simulink library "PDECharactLib"  (R2019a)
settings: Solver=VariableStepAuto  StartTime=0.0  StopTime=10.0  RelTol=1e-3
settings Model: Creator=User  LastModifiedBy=kc5492

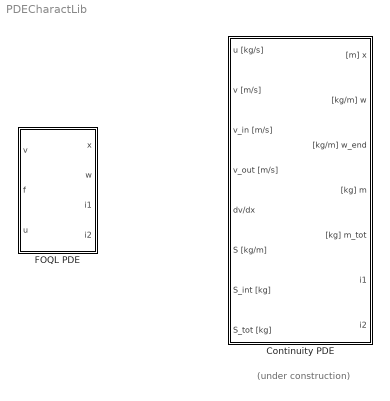
== system PDECharactLib ==
  note: (under construction)
  Continuity PDE : Subsystem  mask(First-order quasilinear PDE solver){ell=1, Nmax=100, x0=0:0.1:1, w0=1:-0.1:0, m0=0.095:-0.01:0.005, initM_tot=0, initX=0, initW=0, initM=0, dx=0.1, dw=0.1, dt=0.1, crossing_tol=1e-11, overflow_err=off}
      mask prompts: ell "Domain length (L)"; Nmax "Maximum number of characteristics (Nmax)"; x0 "x-values"; w0 "w-values"; m0 "m-values"; initM_tot "total mass"; initX "(hidden) Full initial x"; initW "(hidden) Full initial w"; initM "(hidden) Full initial m"; dx "∆x"; dw "∆w"; dt "∆t"; crossing_tol "Tolerance for crossing characteristics"; overflow_err "Terminate on overflow"
      mask help:
      | Implementation of the method of characteristics for the first-order quasilinear PDE
      |
      | 	∂w(t, x)/∂t + v(t, x) ∂w(t, x)/∂x = f(t, x),    t ≥ 0,    x ∈ [0, L],
      | 	w(0, x) = w0(x),
      | 	w(t, 0) = u(t).
      |
      | The functions v, f, and u are provided through the inputs and can also depend on variables other than time.
      |
      | The number of characteristics to be integrated simultaneously is limited by Nmax. The current number of characteristics is output through the port N.
      |
      | Initial state function w0(x) is defined by its grid values (x, w) which also define the initial set of characteristics. The vector of x-values should be non-decreasing and span from 0 to L. The vector of w-values should be the same length as x-values.
      |
      | If the latest characteristic was created at time t0 and currently passes through the point (x, w) then new characteristic is created at the boundary x = 0 if at least one of the conditions is satisfied:
      |     • x > ∆x,
      |     • |w - u(t)| > ∆w,
      |     • t - t0 > ∆t.
      |
      | Error is thrown when two characteristics intersect with overlap more than that defined as "Tolerance for crossing characteristics" or when the flag "Terminate on overflow" is set and the number of characteristics exceeds Nmax.
      mask init:
      | initX = [x0, zeros(1, Nmax-length(x0))];
      | initW = [w0, zeros(1, Nmax-length(w0))];
      | initM = [0, m0, zeros(1, Nmax-length(m0)-1)];
      mask DialogControl Container4 Prompt: Initial state
      mask DialogControl Container3 Prompt: Conditions for creating a new characteristic
  FOQL PDE : Subsystem  mask(First-order quasilinear PDE solver){ell=1, Nmax=100, x0=0:0.1:1, w0=(0:0.1:1).^2, initX=0, initW=0, dx=0.1, dw=0.1, dt=0.1, crossing_tol=1e-11, overflow_err=off}
      mask prompts: ell "Domain length (L)"; Nmax "Maximum number of characteristics (Nmax)"; x0 "x-values"; w0 "w-values"; initX "(hidden) Full initial x"; initW "(hidden) Full initial w"; dx "∆x"; dw "∆w"; dt "∆t"; crossing_tol "Tolerance for crossing characteristics"; overflow_err "Terminate on overflow"
      mask help:
      | Implementation of the method of characteristics for the first-order quasilinear PDE
      |
      | 	∂w(t, x)/∂t + v(t, x) ∂w(t, x)/∂x = f(t, x),    t ≥ 0,    x ∈ [0, L],
      | 	w(0, x) = w0(x),
      | 	w(t, 0) = u(t).
      |
      | The functions v, f, and u are provided through the inputs and can also depend on variables other than time.
      |
      | The number of characteristics to be integrated simultaneously is limited by Nmax. The current number of characteristics is output through the port N.
      |
      | Initial state function w0(x) is defined by its grid values (x, w) which also define the initial set of characteristics. The vector of x-values should be non-decreasing and span from 0 to L. The vector of w-values should be the same length as x-values.
      |
      | If the latest characteristic was created at time t0 and currently passes through the point (x, w) then new characteristic is created at the boundary x = 0 if at least one of the conditions is satisfied:
      |     • x > ∆x,
      |     • |w - u(t)| > ∆w,
      |     • t - t0 > ∆t.
      |
      | Error is thrown when two characteristics intersect with overlap more than that defined as "Tolerance for crossing characteristics" or when the flag "Terminate on overflow" is set and the number of characteristics exceeds Nmax.
      mask init:
      | initX = [x0, zeros(1, Nmax-length(x0))];
      | initW = [w0, zeros(1, Nmax-length(w0))];
      mask DialogControl Container4 Prompt: Initial state
      mask DialogControl Container3 Prompt: Conditions for creating a new characteristic

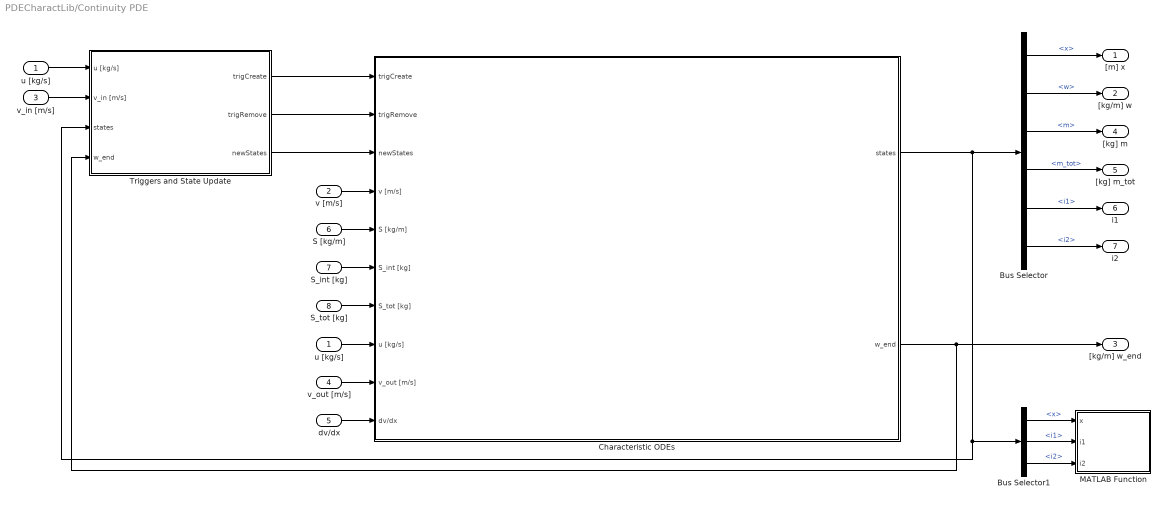
== system PDECharactLib/Continuity PDE ==
  u [kg/s] : Inport
  v [m/s] : Inport  Port=2
  v_in [m/s] : Inport  Port=3
  v_out [m/s] : Inport  Port=4
  dv/dx : Inport  Port=5
  S [kg/m] : Inport  Port=6
  S_int [kg] : Inport  Port=7
  S_tot [kg] : Inport  Port=8
  " u [kg/s] " : InportShadow
  Bus Selector : BusSelector  OutputSignals=x,w,m,m_tot,i1,i2
  Bus Selector1 : BusSelector  OutputSignals=x,i1,i2
  Characteristic ODEs : Subsystem
  MATLAB Function : MATLAB Function  TreatAsAtomicUnit=on
  Triggers and State Update : Subsystem
  "[m] x" : Outport
  "[kg/m] w" : Outport  Port=2
  "[kg/m] w_end" : Outport  Port=3
  "[kg] m" : Outport  Port=4
  "[kg] m_tot" : Outport  Port=5
  i1 : Outport  Port=6
  i2 : Outport  Port=7
  wires:
  u [kg/s]/1 -> Triggers and State Update/1(u [kg/s])
  v [m/s]/1 -> Characteristic ODEs/4(v [m/s])
  Triggers and State Update/1(trigCreate) -> Characteristic ODEs/1(trigCreate)
  Triggers and State Update/2(trigRemove) -> Characteristic ODEs/2(trigRemove)
  S [kg/m]/1 -> Characteristic ODEs/5(S [kg/m])
  S_int [kg]/1 -> Characteristic ODEs/6(S_int [kg])
  S_tot [kg]/1 -> Characteristic ODEs/7(S_tot [kg])
  " u [kg/s] "/1 -> Characteristic ODEs/8(u [kg/s])
  v_out [m/s]/1 -> Characteristic ODEs/9(v_out [m/s])
  dv/dx/1 -> Characteristic ODEs/10(dv/dx)
  Triggers and State Update/3(newStates) -> Characteristic ODEs/3(newStates)
  Characteristic ODEs/1(states) -> Triggers and State Update/3(states), Bus Selector1/1, Bus Selector/1
  Characteristic ODEs/2(w_end) -> Triggers and State Update/4(w_end), "[kg/m] w_end"/1
  Bus Selector/1 -> "[m] x"/1  "<x>"
  Bus Selector/2 -> "[kg/m] w"/1  "<w>"
  Bus Selector/3 -> "[kg] m"/1  "<m>"
  Bus Selector/4 -> "[kg] m_tot"/1  "<m_tot>"
  Bus Selector/5 -> i1/1  "<i1>"
  Bus Selector/6 -> i2/1  "<i2>"
  Bus Selector1/1 -> MATLAB Function/1(x)  "<x>"
  Bus Selector1/2 -> MATLAB Function/2(i1)  "<i1>"
  Bus Selector1/3 -> MATLAB Function/3(i2)  "<i2>"
  v_in [m/s]/1 -> Triggers and State Update/2(v_in [m/s])

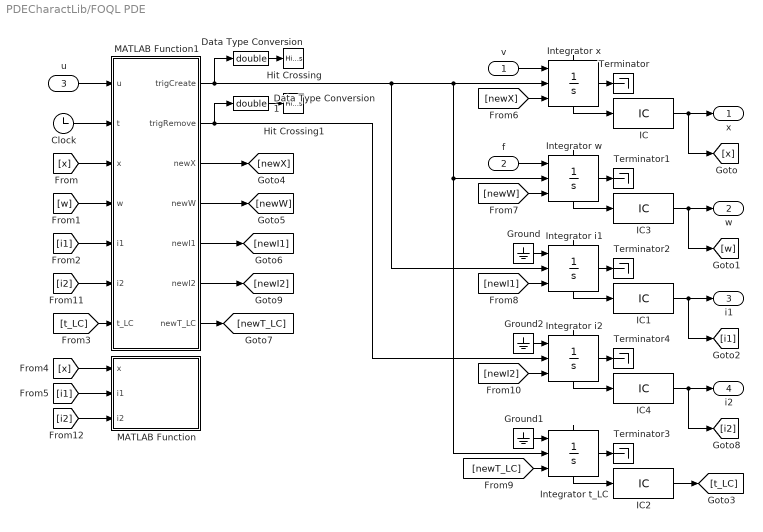
== system PDECharactLib/FOQL PDE ==
  v : Inport
  f : Inport  Port=2
  u : Inport  Port=3
  Clock : Clock
  Data Type Conversion : DataTypeConversion  OutDataTypeStr=double
  Data Type Conversion1 : DataTypeConversion  OutDataTypeStr=double
  Ground : Ground
  Ground1 : Ground
  Ground2 : Ground
  Hit Crossing : HitCross  ShowOutputPort=off
  Hit Crossing1 : HitCross  ShowOutputPort=off
  IC : InitialCondition  Value=initX
  IC1 : InitialCondition
  IC2 : InitialCondition  Value=0
  IC3 : InitialCondition  Value=initW
  IC4 : InitialCondition  Value=length(x0)
  Integrator i1 : Integrator  ExternalReset=level hold  InitialConditionSource=external  InitialCondition=[length(x0); 0]  ShowStatePort=on
  Integrator i2 : Integrator  ExternalReset=level hold  InitialConditionSource=external  InitialCondition=[length(x0); 0]  ShowStatePort=on
  Integrator t_LC : Integrator  ExternalReset=level hold  InitialConditionSource=external  InitialCondition=[length(x0); 0]  ShowStatePort=on
  Integrator w : Integrator  ExternalReset=level hold  InitialConditionSource=external  ShowStatePort=on
  Integrator x : Integrator  ExternalReset=level hold  InitialConditionSource=external  ShowStatePort=on
  MATLAB Function : MATLAB Function  TreatAsAtomicUnit=on
  MATLAB Function1 : MATLAB Function  TreatAsAtomicUnit=on
  Terminator{,1..4} (5 alike) : Terminator
  x : Outport
  w : Outport  Port=2
  i1 : Outport  Port=3
  i2 : Outport  Port=4
  wires:
  Integrator x/State -> IC/1
  u/1 -> MATLAB Function1/1(u)
  Clock/1 -> MATLAB Function1/2(t)
  Integrator i1/State -> IC1/1
  Integrator t_LC/State -> IC2/1
  MATLAB Function1/1(trigCreate) -> Integrator w/2, Integrator t_LC/2, Integrator x/2, Integrator i1/2, Data Type Conversion/1
  Data Type Conversion/1 -> Hit Crossing/1
  Data Type Conversion1/1 -> Hit Crossing1/1
  IC/1 -> x/1, [x]
  IC3/1 -> w/1, [w]
  Integrator w/State -> IC3/1
  v/1 -> Integrator x/1
  f/1 -> Integrator w/1
  IC1/1 -> i1/1, [i1]
  Ground/1 -> Integrator i1/1
  Ground1/1 -> Integrator t_LC/1
  Integrator x/1 -> Terminator/1
  Integrator w/1 -> Terminator1/1
  Integrator i1/1 -> Terminator2/1
  Integrator t_LC/1 -> Terminator3/1
  IC2/1 -> [t_LC]
  MATLAB Function1/3(newX) -> [newX]
  MATLAB Function1/4(newW) -> [newW]
  MATLAB Function1/5(newI1) -> [newI1]
  MATLAB Function1/7(newT_LC) -> [newT_LC]
  MATLAB Function1/2(trigRemove) -> Integrator i2/2, Data Type Conversion1/1
  [newT_LC] -> Integrator t_LC/3
  [newX] -> Integrator x/3
  [newW] -> Integrator w/3
  [newI1] -> Integrator i1/3
  [x] -> MATLAB Function/1(x)
  [i1] -> MATLAB Function/2(i1)
  [t_LC] -> MATLAB Function1/7(t_LC)
  [i1] -> MATLAB Function1/5(i1)
  [w] -> MATLAB Function1/4(w)
  [x] -> MATLAB Function1/3(x)
  [newI2] -> Integrator i2/3
  Integrator i2/1 -> Terminator4/1
  IC4/1 -> [i2], i2/1
  Integrator i2/State -> IC4/1
  Ground2/1 -> Integrator i2/1
  [i2] -> MATLAB Function1/6(i2)
  [i2] -> MATLAB Function/3(i2)
  MATLAB Function1/6(newI2) -> [newI2]

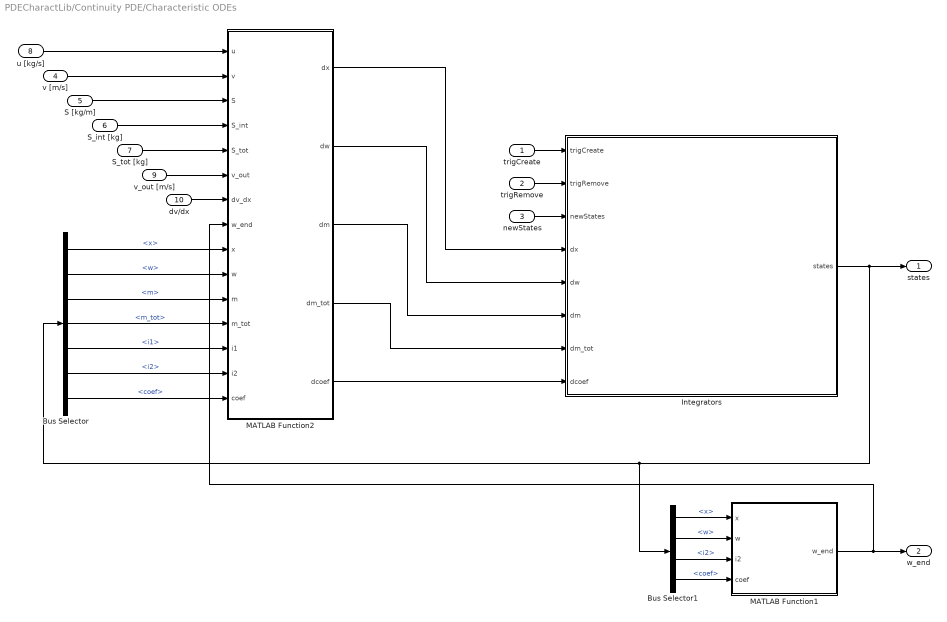
== system PDECharactLib/Continuity PDE/Characteristic ODEs ==
  trigCreate : Inport
  trigRemove : Inport  Port=2
  newStates : Inport  Port=3
  v [m/s] : Inport  Port=4
  S [kg/m] : Inport  Port=5
  S_int [kg] : Inport  Port=6
  S_tot [kg] : Inport  Port=7
  u [kg/s] : Inport  Port=8
  v_out [m/s] : Inport  Port=9
  dv/dx : Inport  Port=10
  Bus Selector : BusSelector  OutputSignals=x,w,m,m_tot,i1,i2,coef
  Bus Selector1 : BusSelector  OutputSignals=x,w,i2,coef
  Integrators : Subsystem
  MATLAB Function1 : MATLAB Function  TreatAsAtomicUnit=on
  MATLAB Function2 : MATLAB Function  TreatAsAtomicUnit=on
  states : Outport
  w_end : Outport  Port=2
  wires:
  S [kg/m]/1 -> MATLAB Function2/3(S)
  v_out [m/s]/1 -> MATLAB Function2/6(v_out)
  u [kg/s]/1 -> MATLAB Function2/1(u)
  S_tot [kg]/1 -> MATLAB Function2/5(S_tot)
  trigRemove/1 -> Integrators/2(trigRemove)
  dv/dx/1 -> MATLAB Function2/7(dv_dx)
  S_int [kg]/1 -> MATLAB Function2/4(S_int)
  trigCreate/1 -> Integrators/1(trigCreate)
  MATLAB Function2/2(dw) -> Integrators/5(dw)
  MATLAB Function2/3(dm) -> Integrators/6(dm)
  MATLAB Function2/4(dm_tot) -> Integrators/7(dm_tot)
  MATLAB Function2/5(dcoef) -> Integrators/8(dcoef)
  newStates/1 -> Integrators/3(newStates)
  Integrators/1(states) -> Bus Selector/1, Bus Selector1/1, states/1
  Bus Selector/1 -> MATLAB Function2/9(x)  "<x>"
  Bus Selector/2 -> MATLAB Function2/10(w)  "<w>"
  Bus Selector/5 -> MATLAB Function2/13(i1)  "<i1>"
  Bus Selector/6 -> MATLAB Function2/14(i2)  "<i2>"
  v [m/s]/1 -> MATLAB Function2/2(v)
  MATLAB Function1/1(w_end) -> MATLAB Function2/8(w_end), w_end/1
  Bus Selector1/1 -> MATLAB Function1/1(x)  "<x>"
  Bus Selector1/2 -> MATLAB Function1/2(w)  "<w>"
  Bus Selector1/3 -> MATLAB Function1/3(i2)  "<i2>"
  Bus Selector1/4 -> MATLAB Function1/4(coef)  "<coef>"
  Bus Selector/7 -> MATLAB Function2/15(coef)  "<coef>"
  Bus Selector/4 -> MATLAB Function2/12(m_tot)  "<m_tot>"
  Bus Selector/3 -> MATLAB Function2/11(m)  "<m>"
  MATLAB Function2/1(dx) -> Integrators/4(dx)

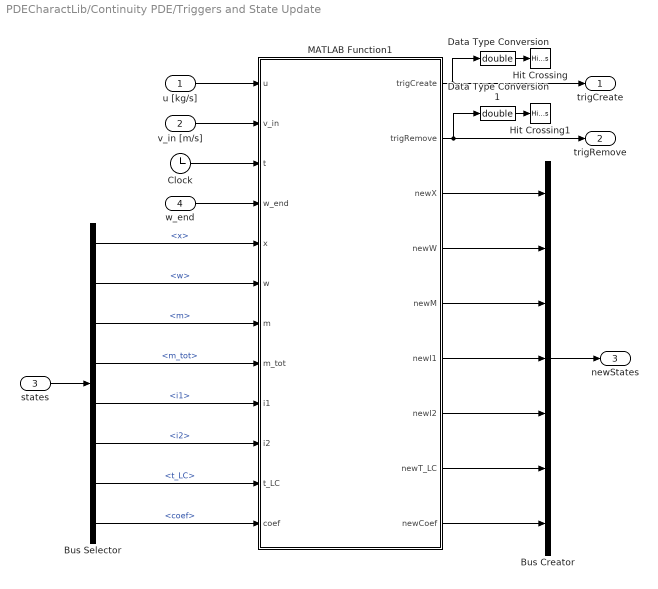
== system PDECharactLib/Continuity PDE/Triggers and State Update ==
  u [kg/s] : Inport
  v_in [m/s] : Inport  Port=2
  states : Inport  Port=3
  w_end : Inport  Port=4
  Bus Creator : BusCreator  Inputs=7
  Bus Selector : BusSelector  OutputSignals=x,w,m,m_tot,i1,i2,t_LC,coef
  Clock : Clock
  Data Type Conversion : DataTypeConversion  OutDataTypeStr=double
  Data Type Conversion1 : DataTypeConversion  OutDataTypeStr=double
  Hit Crossing : HitCross  ShowOutputPort=off
  Hit Crossing1 : HitCross  ShowOutputPort=off
  MATLAB Function1 : MATLAB Function  TreatAsAtomicUnit=on
  trigCreate : Outport
  trigRemove : Outport  Port=2
  newStates : Outport  Port=3
  wires:
  Data Type Conversion1/1 -> Hit Crossing1/1
  MATLAB Function1/2(trigRemove) -> trigRemove/1, Data Type Conversion1/1
  Clock/1 -> MATLAB Function1/3(t)
  MATLAB Function1/3(newX) -> Bus Creator/1
  u [kg/s]/1 -> MATLAB Function1/1(u)
  Data Type Conversion/1 -> Hit Crossing/1
  MATLAB Function1/1(trigCreate) -> trigCreate/1, Data Type Conversion/1
  MATLAB Function1/4(newW) -> Bus Creator/2
  w_end/1 -> MATLAB Function1/4(w_end)
  Bus Creator/1 -> newStates/1
  MATLAB Function1/5(newM) -> Bus Creator/3
  MATLAB Function1/6(newI1) -> Bus Creator/4
  MATLAB Function1/7(newI2) -> Bus Creator/5
  MATLAB Function1/8(newT_LC) -> Bus Creator/6
  states/1 -> Bus Selector/1
  Bus Selector/1 -> MATLAB Function1/5(x)  "<x>"
  Bus Selector/8 -> MATLAB Function1/12(coef)  "<coef>"
  Bus Selector/7 -> MATLAB Function1/11(t_LC)  "<t_LC>"
  Bus Selector/6 -> MATLAB Function1/10(i2)  "<i2>"
  Bus Selector/5 -> MATLAB Function1/9(i1)  "<i1>"
  Bus Selector/3 -> MATLAB Function1/7(m)  "<m>"
  Bus Selector/2 -> MATLAB Function1/6(w)  "<w>"
  MATLAB Function1/9(newCoef) -> Bus Creator/7
  Bus Selector/4 -> MATLAB Function1/8(m_tot)  "<m_tot>"
  v_in [m/s]/1 -> MATLAB Function1/2(v_in)

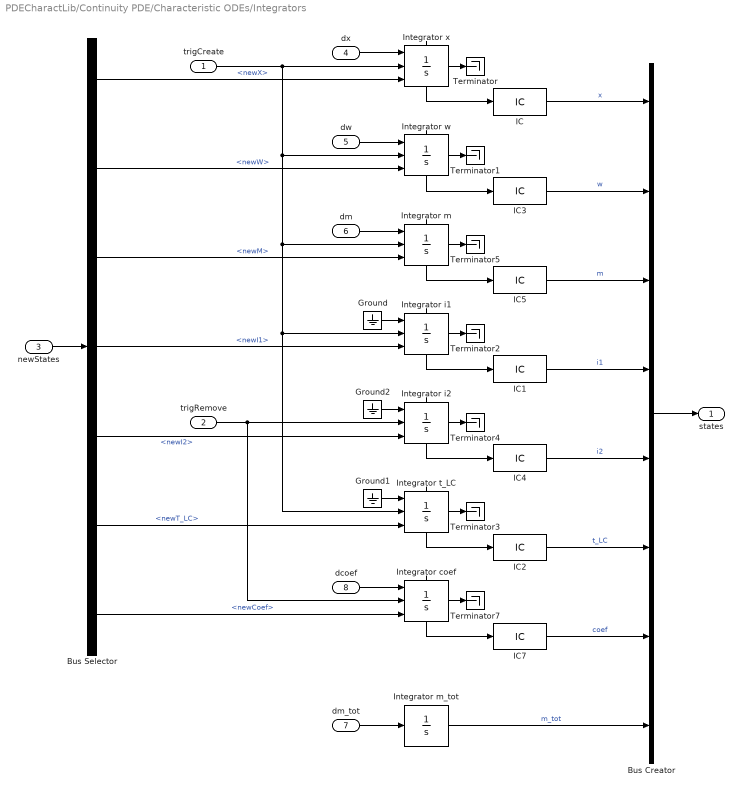
== system PDECharactLib/Continuity PDE/Characteristic ODEs/Integrators ==
  trigCreate : Inport
  trigRemove : Inport  Port=2
  newStates : Inport  Port=3
  dx : Inport  Port=4
  dw : Inport  Port=5
  dm : Inport  Port=6
  dm_tot : Inport  Port=7
  dcoef : Inport  Port=8
  Bus Creator : BusCreator  Inputs=8
  Bus Selector : BusSelector  OutputSignals=newX,newW,newM,newI1,newI2,newT_LC,newCoef
  Ground : Ground
  Ground1 : Ground
  Ground2 : Ground
  IC : InitialCondition  Value=initX
  IC1 : InitialCondition
  IC2 : InitialCondition  Value=0
  IC3 : InitialCondition  Value=initW
  IC4 : InitialCondition  Value=length(x0)
  IC5 : InitialCondition  Value=initM
  IC7 : InitialCondition  Value=[0 0]
  Integrator coef : Integrator  ExternalReset=level hold  InitialConditionSource=external  InitialCondition=[length(x0); 0]  ShowStatePort=on
  Integrator i1 : Integrator  ExternalReset=level hold  InitialConditionSource=external  InitialCondition=[length(x0); 0]  ShowStatePort=on
  Integrator i2 : Integrator  ExternalReset=level hold  InitialConditionSource=external  InitialCondition=[length(x0); 0]  ShowStatePort=on
  Integrator m : Integrator  ExternalReset=level hold  InitialConditionSource=external  InitialCondition=[length(x0); 0]  ShowStatePort=on
  Integrator m_tot : Integrator  InitialCondition=initM_tot
  Integrator t_LC : Integrator  ExternalReset=level hold  InitialConditionSource=external  InitialCondition=[length(x0); 0]  ShowStatePort=on
  Integrator w : Integrator  ExternalReset=level hold  InitialConditionSource=external  ShowStatePort=on
  Integrator x : Integrator  ExternalReset=level hold  InitialConditionSource=external  ShowStatePort=on
  Terminator{,1..5,7} (7 alike) : Terminator
  states : Outport
  wires:
  Integrator coef/State -> IC7/1
  Integrator m/1 -> Terminator5/1
  trigCreate/1 -> Integrator x/2, Integrator t_LC/2, Integrator i1/2, Integrator m/2, Integrator w/2
  Integrator coef/1 -> Terminator7/1
  trigRemove/1 -> Integrator coef/2, Integrator i2/2
  Ground2/1 -> Integrator i2/1
  Ground1/1 -> Integrator t_LC/1
  Integrator i2/State -> IC4/1
  Integrator i1/1 -> Terminator2/1
  Integrator w/State -> IC3/1
  Integrator x/1 -> Terminator/1
  Integrator t_LC/1 -> Terminator3/1
  dx/1 -> Integrator x/1
  Integrator t_LC/State -> IC2/1
  Integrator w/1 -> Terminator1/1
  Integrator i1/State -> IC1/1
  Ground/1 -> Integrator i1/1
  Integrator x/State -> IC/1
  Integrator i2/1 -> Terminator4/1
  Integrator m/State -> IC5/1
  dw/1 -> Integrator w/1
  dm/1 -> Integrator m/1
  dm_tot/1 -> Integrator m_tot/1
  dcoef/1 -> Integrator coef/1
  newStates/1 -> Bus Selector/1
  Bus Selector/1 -> Integrator x/3  "<newX>"
  Bus Selector/2 -> Integrator w/3  "<newW>"
  Bus Selector/3 -> Integrator m/3  "<newM>"
  Bus Selector/5 -> Integrator i2/3  "<newI2>"
  Bus Selector/6 -> Integrator t_LC/3  "<newT_LC>"
  Bus Selector/7 -> Integrator coef/3  "<newCoef>"
  IC7/1 -> Bus Creator/7  "coef"
  IC2/1 -> Bus Creator/6  "t_LC"
  IC4/1 -> Bus Creator/5  "i2"
  IC1/1 -> Bus Creator/4  "i1"
  Integrator m_tot/1 -> Bus Creator/8  "m_tot"
  IC5/1 -> Bus Creator/3  "m"
  IC3/1 -> Bus Creator/2  "w"
  IC/1 -> Bus Creator/1  "x"
  Bus Creator/1 -> states/1
  Bus Selector/4 -> Integrator i1/3  "<newI1>"

== matlab function PDECharactLib/Continuity PDE/MATLAB Function ==
  data: x input size=Nmax; i1 input size=1; i2 input size=1; crossing_tol parameter size=1; Nmax parameter size=1
function checkCross(x, i1, i2, crossing_tol, Nmax)

if i1 < i2
    ind = i1:i2;
else
    ind = [i1:Nmax, 1:i2];
end

if length(ind) > 1 && any(x(ind(1:end-1)) - x(ind(2:end)) >= crossing_tol)
    error('Crossing characteristics detected with tolerance %f.', crossing_tol);
end

== matlab function PDECharactLib/Continuity PDE/Triggers and State Update/MATLAB Function1 ==
  data: u input size=1; v_in input; t input size=1; w_end input size=1; x input size=Nmax; w input size=Nmax; m input size=Nmax; m_tot input size=1; i1 input size=1; i2 input size=1; t_LC input size=1; coef input size=2; trigCreate output boolean size=1; trigRemove output boolean size=1; newX output size=Nmax; newW output size=Nmax; newM output size=Nmax; newI1 output size=1; newI2 output size=1; newT_LC output size=1; dx parameter size=1; dw parameter size=1; dt parameter size=1; Nmax parameter size=1; overflow_err parameter size=1; ell parameter size=1; newCoef output size=2
function [trigCreate, trigRemove, newX, newW, newM, newI1, newI2, newT_LC, newCoef] = ...
    updateState(u, v_in, t, w_end, x, w, m, m_tot, i1, i2, t_LC, coef, dx, dw, dt, Nmax, overflow_err, ell)

if i1 < i2
    ind = i1:i2;
else
    ind = [i1:Nmax, 1:i2];
end

trigRemove = (length(ind) > 1) && (x(i2) >= ell);
trigCreate = (x(i1) >= dx) || ...
             (abs(w(i1)-u) >= dw) || ...
             (t-t_LC >= dt);

if trigRemove
    ind = ind(1:end-1);
    newI2 = ind(end);
    z = ell - x(newI2);
    m_rem = m_tot - sum(m(ind));
    A = [0, 0, 1; z^2, z, 1; z^3/3, z^2/2, z];
    b = [w(newI2); w_end; m_rem];
    newCoef = eye(2,3)*(A\b);
else
    newI2 = i2;
    newCoef = coef;
end

newX = x;
newW = w;
newM = m;
if trigCreate && (length(ind) < Nmax)
    % create characteristic
    newI1 = mod(i1-2, Nmax) + 1;
    newX(newI1) = 0;
    newW(newI1) = u/v_in;
    newM(newI1) = 0;
    newT_LC = t;
elseif trigCreate && (length(ind) == Nmax) && overflow_err
    error('Maximum number of characteristics (%d) is exceeded.', Nmax);
else
    newI1 = i1;
    newT_LC = t_LC;
    trigCreate = false;
end

== matlab function PDECharactLib/Continuity PDE/Characteristic ODEs/MATLAB Function2 ==
  data: u input size=1; v input size=Nmax; dx output size=Nmax; S input size=Nmax; S_int input size=Nmax; S_tot input size=1; v_out input size=1; dv_dx input size=Nmax; w_end input size=1; dw output size=Nmax; dm output size=Nmax; dm_tot output size=1; x input size=Nmax; w input size=Nmax; m input size=Nmax; m_tot input size=1; i1 input size=1; i2 input size=1; coef input size=2; dcoef output size=2; ell parameter size=1
function [dx, dw, dm, dm_tot, dcoef] = derivatives(u, v, S, S_int, S_tot, v_out, dv_dx, w_end, x, w, m, m_tot, i1, i2, coef, ell)

dx = v;

dw = S - dv_dx .* w;

dm = S_int;
dm(i1) = dm(i1) + u;

dm_tot = S_tot + u - v_out*w_end;

if i1 < i2
    ind = i1:i2;
else
    ind = [i1:length(x), 1:i2];
end

m_rem = m_tot - sum(m(ind));
z = ell - x(i2);
A = [z^3/3, z^2/2; -z^2/2, z^3/3];
c = 0;
b = [-c*([z^3/3, z^2/2, z]*[coef; w(i2)] - m_rem) + S_tot + (v(i2) - v_out)*w_end - z*dw(i2); 0];
dcoef = A\b;

== matlab function PDECharactLib/Continuity PDE/Characteristic ODEs/MATLAB Function1 ==
  data: x input size=Nmax; w input size=Nmax; w_end output size=1; i2 input size=1; coef input size=2; ell parameter size=1
function w_end = calcW_end(x, w, i2, coef, ell)

z = ell - x(i2);
w_end = [z^2, z, 1]*[coef; w(i2)];

== matlab function PDECharactLib/FOQL PDE/MATLAB Function ==
  data: x input; i1 input; i2 input; crossing_tol parameter; Nmax parameter size=1
function checkCross(x, i1, i2, crossing_tol, Nmax)

if i1 < i2
    ind = i1:i2;
else
    ind = [i1:Nmax, 1:i2];
end

if any(x(ind(1:end-1)) - x(ind(2:end)) >= crossing_tol)
    error('Crossing characteristics detected with tolerance %f.', crossing_tol);
end

== matlab function PDECharactLib/FOQL PDE/MATLAB Function1 ==
  data: u input size=1; t input size=1; x input size=Nmax; w input size=Nmax; i1 input size=1; i2 input size=1; t_LC input size=1; trigCreate output size=1; trigRemove output size=1; newX output size=Nmax; newW output size=Nmax; newI1 output size=1; newI2 output size=1; newT_LC output size=1; dx parameter size=1; dw parameter size=1; dt parameter size=1; Nmax parameter size=1; overflow_err parameter size=1; ell parameter size=1
function [trigCreate, trigRemove, newX, newW, newI1, newI2, newT_LC] = ...
    updateState(u, t, x, w, i1, i2, t_LC, dx, dw, dt, Nmax, overflow_err, ell)

if i1 < i2
    ind = i1:i2;
else
    ind = [i1:Nmax, 1:i2];
end

trigRemove = (length(ind) > 2) && (x(ind(end-1)) >= ell);
trigCreate = (x(i1) >= dx) || ...
             (abs(w(i1)-u) >= dw) || ...
             (t-t_LC >= dt);

if trigRemove
    % reduce N
    i = length(ind)-2;
    while (i >= 2) && (x(ind(i)) > ell)
        i = i-1;
    end
    ind = ind(1:i+1);
    newI2 = ind(end);
else
    newI2 = i2;
end

newX = x;
newW = w;
if trigCreate && (length(ind) < Nmax)
    % create characteristic
    newI1 = mod(i1-2, Nmax) + 1;
    newX(newI1) = 0;
    newW(newI1) = u;
    newT_LC = t;
elseif trigCreate && (length(ind) == Nmax) && overflow_err
    error('Maximum number of characteristics (%d) is exceeded.', Nmax);
else
    newI1 = i1;
    newT_LC = t_LC;
    trigCreate = false;
end
